simulink library "motor_lib"  (R2022b)
settings: Solver=VariableStepAuto  StartTime=0.0  StopTime=10.0  RelTol=1e-3
undefined symbols (not defined in the file): raptor_xcp_function
libraries: Raptor_lib x1
settings Model: Creator=serga  LastModifiedBy=serga

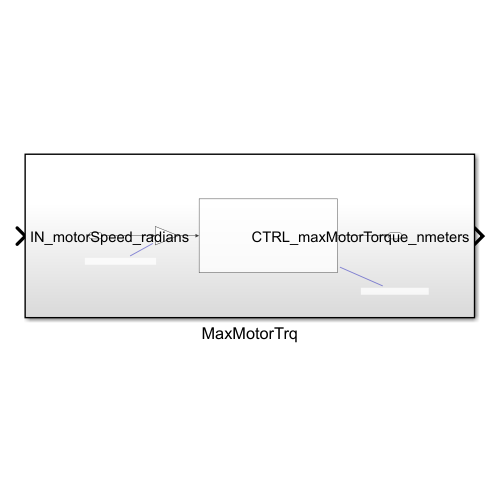
[thumbnail: Simulink's stored preview of the top-level diagram]
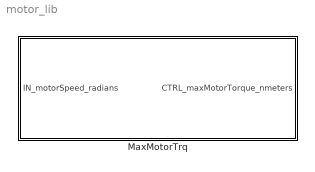
== system motor_lib ==
  MaxMotorTrq : Subsystem

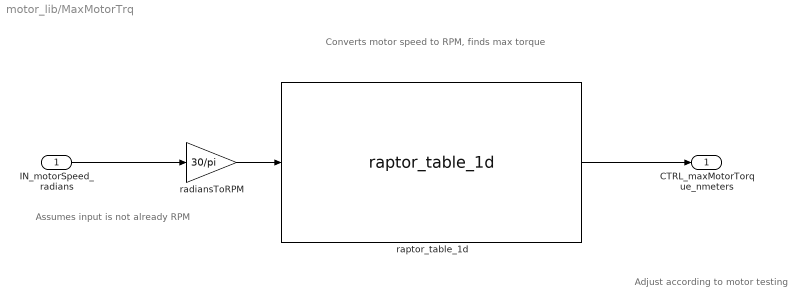
== system motor_lib/MaxMotorTrq ==
  note: Adjust according to motor testing
  note: Assumes input is not already RPM
  note: Converts motor speed to RPM, finds max torque
  IN_motorSpeed_radians : Inport
  radiansToRPM : Gain  Gain=30/pi
  raptor_table_1d : Raptor_lib/Table Lookup/raptor_table_1d  dataName='motorSpeedToMaxMotorTorque'  initValue=[240 240 240 240 240 240 240 240 240 240 240 239 238 237 236 235 234 232 230 229 228 225 223 220 217 215]  dataType=single  storage=Calibration  initValueX=[0 200 400 600 800 1000 1200 1400 1600 1800 2000 2200 2400 2600 2800 3000 3200 3400 3600 3800 4000 4200 4400 4600 4800 5000]  dataTypeXY=single  storageXY=Calibration  calVisible=on  showTable=on  calGain=1.0  calOffset=0.0  calMax=Inf  calMin=-Inf  calFormat='-1'  calUnit='Nm'  calHelp=''  showBreakpoint=on  dataNameX=[]  calGainX=1.0  calOffsetX=0.0  calMaxX=Inf  calMinX=-Inf  calFormatX='-1'  calUnitX='RPM'  calHelpX=''  calAccess=1  calFunction=raptor_xcp_function(gcb)  measureEnable=off  mName=['Data1D_Output']
      settings: SourceProductName=Raptor
  CTRL_maxMotorTorque_nmeters : Outport
  wires:
  IN_motorSpeed_radians/1 -> radiansToRPM/1
  radiansToRPM/1 -> raptor_table_1d/1
  raptor_table_1d/1 -> CTRL_maxMotorTorque_nmeters/1
